simulink model "bug3"  (R2021b)
settings: Solver=VariableStepAuto  StartTime=0.0  StopTime=10.0  RelTol=1e-3
undefined symbols (not defined in the file): Newton, Raphson
libraries: simulink x4
settings Model: SimulationMode=accelerator  PauseTimes=0.2  Creator=user  LastModifiedBy=cemery

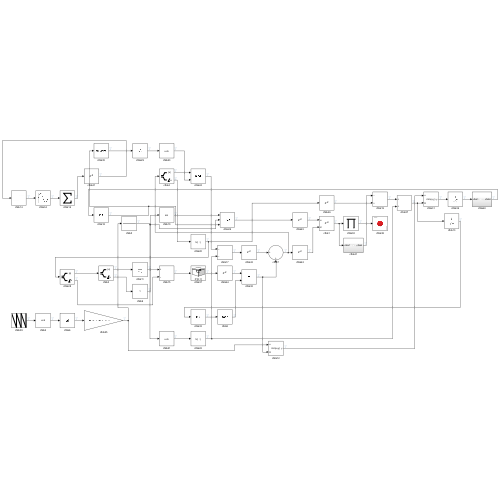
[thumbnail: Simulink's stored preview of the top-level diagram]
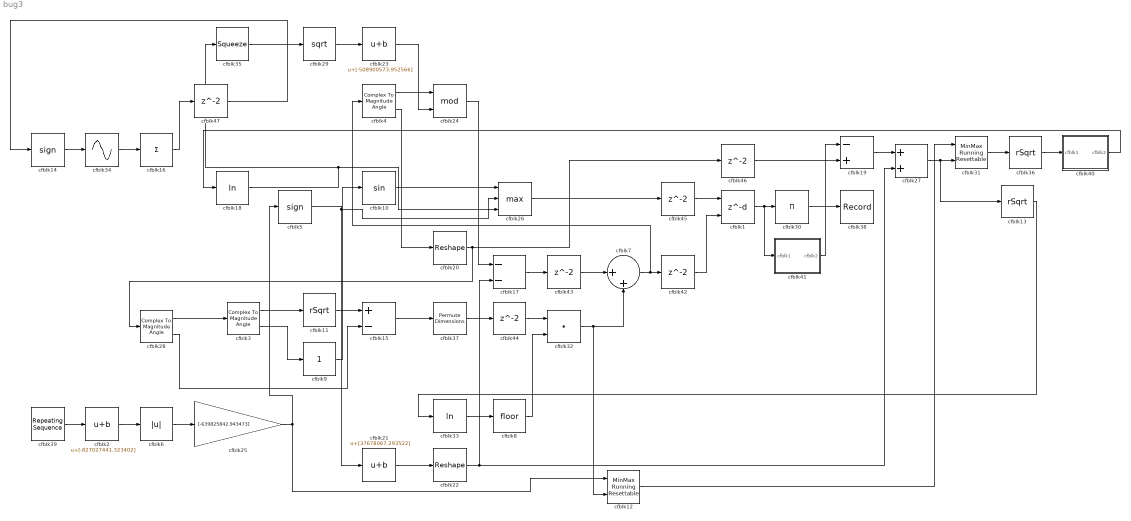
== system bug3 ==
  cfblk1 : Delay  DelayLengthSource=Input port  SampleTime=1
      settings: InputPortMap=u0,p1
  cfblk10 : Trigonometry
  cfblk11 : Sqrt  Operator=rSqrt  AlgorithmType=Newton-Raphson  SaturateOnIntegerOverflow=on
  cfblk12 : simulink/Math Operations/MinMax Running Resettable  Function=min  vinit=0.0
  cfblk13 : Sqrt  Operator=rSqrt  AlgorithmType=Newton-Raphson  SaturateOnIntegerOverflow=on
  cfblk14 : Signum
  cfblk15 : Sum  Inputs=+-
  cfblk16 : Sum  Inputs=+
  cfblk17 : Sum  Inputs=--
  cfblk18 : Math  Operator=log  SaturateOnIntegerOverflow=on
  cfblk19 : Sum  Inputs=-+
  cfblk2 : Bias  Bias=[-827027441.323402]
  cfblk20 : Reshape
  cfblk21 : Bias  Bias=[37678067.293522]
  cfblk22 : Reshape
  cfblk23 : Bias  Bias=[-508900573.952566]
  cfblk24 : Math  Operator=mod  SaturateOnIntegerOverflow=on
  cfblk25 : Gain  Gain=[-639825842.943473]
  cfblk26 : MinMax  Function=max  Inputs=3
  cfblk27 : Sum
  cfblk28 : ComplexToMagnitudeAngle
  cfblk29 : Sqrt  SaturateOnIntegerOverflow=on
  cfblk3 : ComplexToMagnitudeAngle
  cfblk30 : Product  Inputs=*
  cfblk31 : simulink/Math Operations/MinMax Running Resettable  Function=min  vinit=0.0
  cfblk32 : DotProduct  InputSameDT=on  OutDataTypeStr=Inherit: Inherit via internal rule
  cfblk33 : Math  Operator=log  SaturateOnIntegerOverflow=on
  cfblk34 : Sin  TimeSource=Use external signal  SampleTime=0
  cfblk35 : Squeeze
  cfblk36 : Sqrt  Operator=rSqrt  AlgorithmType=Newton-Raphson  SaturateOnIntegerOverflow=on
  cfblk37 : PermuteDimensions
  cfblk38 : Record  FileSettingsInternal="{\"entries\":[{\"content\":{\"excelSettings\":{\"content\":{},\"type\":\"Streamout.ExcelSettings\"}},\"type\":\"Streamout.FileSettingStorage\",\"uuid\":\"430283fb-4cde-40db-b94a-ce57bf0f7a74\"}],\"packageUris\":[\"http://schema.mathworks.com/mf0/streamout_blocks/R2020a\"],\"version\":\"1.0\"}"  SignalsInternal="{\"entries\":[{\"content\":{\"signals\":[{\"content\":{\"blockPath\":[\"sampleModel799_pp_difftest/cfblk38\"],\"channel\":[],\"dimensions\":[1],\"domain\":\"sampleModel799_pp_difftest/cfblk38\",\"lineColor\":\"#22b573\",\"plots\":[1],\"port\":1,\"sid\":[\"\"],\"signalID\":1408,\"signalName\":\"cfblk30\"},\"type\":\"RecordBlkView.Signal\",\"uuid\":\"cdcef453-6688-4cef-b7cc-e70f9411fdb5\"}]},\"type\":\"RecordBlkView.InputSignals\",\"uuid\":\"b4ac560c-f063-4d91-911c-af73cfbdc03d\"}],\"packageUris\":[\"http://schema.mathworks.com/mf0/streamout_blocks/R2020a\"],\"version\":\"1.0\"}"  VisualizationBindings="{\"sparklinesplugin\":{\"info\":[{\"bindingParametersList\":[],\"subplotID\":1}]}}"
  cfblk39 : simulink/Sources/Repeating Sequence  rep_seq_t=[0 2]  rep_seq_y=[902788862.399083, -494348826.288537]
  cfblk4 : ComplexToMagnitudeAngle
  cfblk40 : Subsystem
  cfblk41 : Subsystem
  cfblk{42..47} (6 alike) : Delay  SampleTime=1
  cfblk5 : Signum
  cfblk6 : Abs
  cfblk7 : Sum  Inputs=|++
  cfblk8 : Rounding
  cfblk9 : simulink/Math Operations/Slider Gain  gain=1  low=0  high=2
  wires:
  cfblk37/1 -> cfblk44/1
  cfblk44/1 -> cfblk32/1
  cfblk27/1 -> cfblk13/1, cfblk31/2
  cfblk16/1 -> cfblk47/1
  cfblk47/1 -> cfblk14/1
  cfblk3/1 -> cfblk11/1
  cfblk46/1 -> cfblk19/2
  cfblk43/1 -> cfblk7/1
  cfblk20/1 -> cfblk28/1, cfblk46/1
  cfblk26/1 -> cfblk45/1
  cfblk35/1 -> cfblk29/1
  cfblk45/1 -> cfblk1/1
  cfblk17/1 -> cfblk43/1
  cfblk42/1 -> cfblk1/2
  cfblk28/2 -> cfblk15/2
  cfblk13/1 -> cfblk33/1
  cfblk30/1 -> cfblk38/1
  cfblk10/1 -> cfblk26/1
  cfblk12/1 -> cfblk31/1
  cfblk3/2 -> cfblk9/1
  cfblk19/1 -> cfblk27/1
  cfblk23/1 -> cfblk24/2
  cfblk9/1 -> cfblk10/1
  cfblk4/2 -> cfblk20/1
  cfblk4/1 -> cfblk24/1
  cfblk39/1 -> cfblk2/1
  cfblk8/1 -> cfblk32/2
  cfblk41/1(cfblk2) -> cfblk19/1
  cfblk40/1(cfblk2) -> cfblk18/1
  cfblk11/1 -> cfblk15/1
  cfblk36/1 -> cfblk40/1(cfblk1)
  cfblk28/1 -> cfblk3/1
  cfblk6/1 -> cfblk25/1
  cfblk29/1 -> cfblk23/1
  cfblk25/1 -> cfblk5/1, cfblk12/1
  cfblk24/1 -> cfblk17/1
  cfblk14/1 -> cfblk34/1
  cfblk31/1 -> cfblk36/1
  cfblk15/1 -> cfblk37/1
  cfblk2/1 -> cfblk6/1
  cfblk33/1 -> cfblk8/1
  cfblk21/1 -> cfblk22/1
  cfblk34/1 -> cfblk16/1
  cfblk7/1 -> cfblk4/1, cfblk42/1
  cfblk22/1 -> cfblk17/2, cfblk27/2
  cfblk32/1 -> cfblk7/2, cfblk12/2
  cfblk18/1 -> cfblk35/1, cfblk26/3
  cfblk5/1 -> cfblk21/1, cfblk26/2
  cfblk1/1 -> cfblk30/1, cfblk41/1(cfblk1)

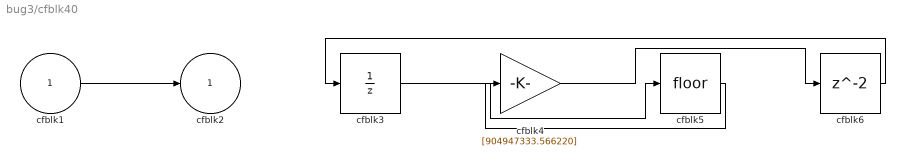
== system bug3/cfblk40 ==
  cfblk1 : Inport
  cfblk3 : UnitDelay  HasFrameUpgradeWarning=on
  cfblk4 : Gain  Gain=[904947333.566220]
  cfblk5 : Rounding
  cfblk6 : Delay  SampleTime=1
  cfblk2 : Outport
  wires:
  cfblk1/1 -> cfblk2/1
  cfblk3/1 -> cfblk5/1
  cfblk5/1 -> cfblk4/1
  cfblk4/1 -> cfblk6/1
  cfblk6/1 -> cfblk3/1

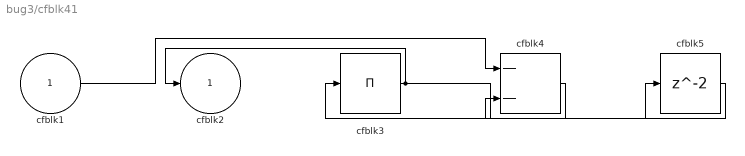
== system bug3/cfblk41 ==
  cfblk1 : Inport
  cfblk3 : Product  Inputs=*
  cfblk4 : Sum  Inputs=--
  cfblk5 : Delay  SampleTime=1
  cfblk2 : Outport
  wires:
  cfblk3/1 -> cfblk2/1, cfblk5/1
  cfblk1/1 -> cfblk4/1
  cfblk4/1 -> cfblk3/1
  cfblk5/1 -> cfblk4/2
